simulink model "control_motor"  (R2024a)
settings: Solver=VariableStepAuto  StartTime=0.0  StopTime=1  FixedStep=0.0001  RelTol=1e-3
libraries: spsMosfetLib x8, spsGroundLib x2, eeTransforms x2, slpidlib x2, spsDCVoltageSourceLib x1, spsStepperMotorLib x1, spsVoltageMeasurementLib x1, spsTriangleGeneratorLib x1, sps_lib x1
settings Model: Creator=Damian  LastModifiedBy=PC
settings SolverCC: MaxConsecutiveZCs=100  MaxConsecutiveMinStep=10000  AllowMultiTaskInputOutput=on  ZeroCrossControl=EnableAll
settings ModelReferenceCC: ModelReferenceMinAlgLoopOccurrences=on

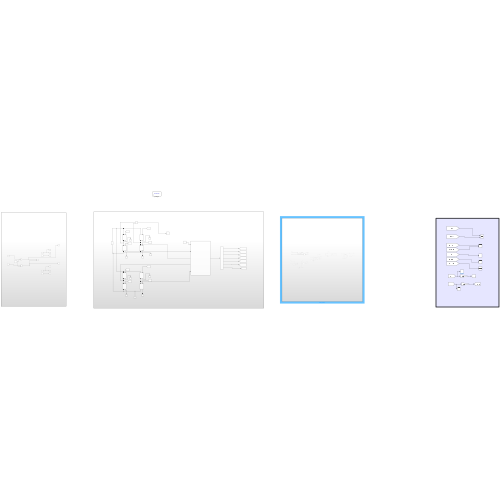
[thumbnail: Simulink's stored preview of the top-level diagram]
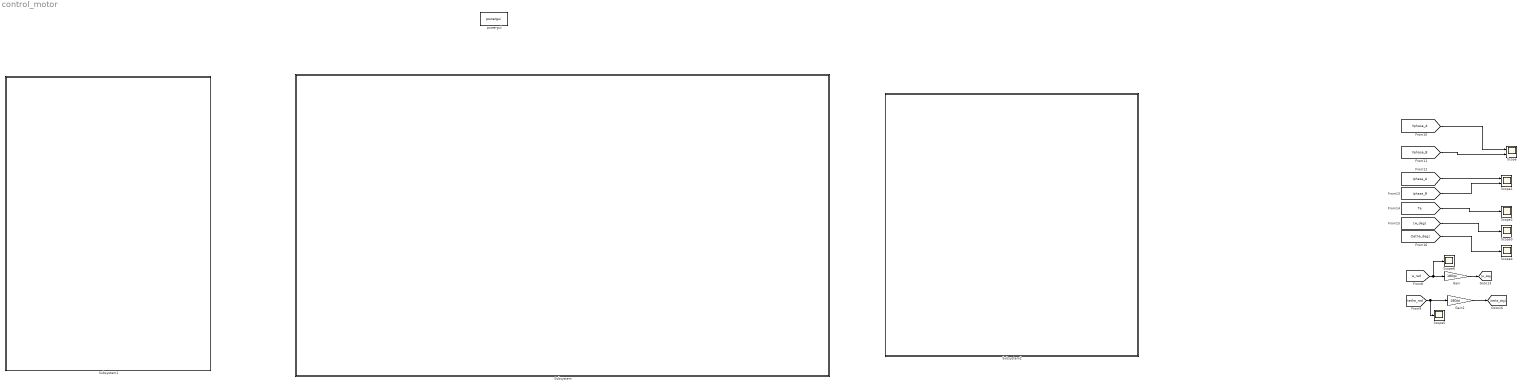
== system control_motor ==
  Gain : Gain  Gain=180/pi
  Gain1 : Gain  Gain=180/pi
  Scope : Scope  NumInputPorts=2
  Scope1 : Scope  NumInputPorts=2
  Scope{2..6} (5 alike) : Scope
  Subsystem : Subsystem
  Subsystem1 : Subsystem
  Subsystem2 : Subsystem
  powergui : sps_lib/powergui  Priority=1  SimulationMode=Continuous  SampleTime=1e-1  frequency=60  Iterations=50  frequencyindice=0  Pbase=100e6  ErrMax=1e-4  UnitsV=kV  UnitsW=MW  buscounter=0  FunctionMessages=off  echomessages=off  EnableUseOfTLC=off  CurrentSourceSwitches=off  DisableSnubberDevices=off  DisableRonSwitches=off  DisableVfSwitches=off  DisplayEquations=off  AutomaticDiscreteSolvers=off  SolverType=Tustin/Backward Euler (TBE)  Interpol=off  ExternalGateDelay=off  methode=off  Ts=100  x0status=blocks  SPID=on  SwTol=0  HookPort=off  NonlinearTolerance=1e-4  nMaxIteration=100  ContinueOnMaxIteration=off  RestoreLinks=warning  ResistiveCurrentMeasurement=off  Frange=[0:2:500]  Ylog=off  Xlog=on  ShowGrid=off  save=off  variable=ZData  structure=0  ZoomFFT=off  StartTime=0.0  cycles=1  DisplayStyle=1  fundamental=60  FreqAxis=off  MaxFrequency=1000  frequencyindicesteady=1  RmsSteady=1  display=off
  wires:
  [w_rad] -> Scope6/1, Gain/1
  Gain/1 -> [w_deg]
  [tetha_rad] -> Scope5/1, Gain1/1
  Gain1/1 -> [tetha_deg]
  [Vphase_A] -> Scope/1
  [Vphase_B] -> Scope/2
  [Iphase_A] -> Scope1/1
  [Iphase_B] -> Scope1/2
  [Te] -> Scope2/1
  [w_deg] -> Scope3/1
  [tetha_deg] -> Scope4/1

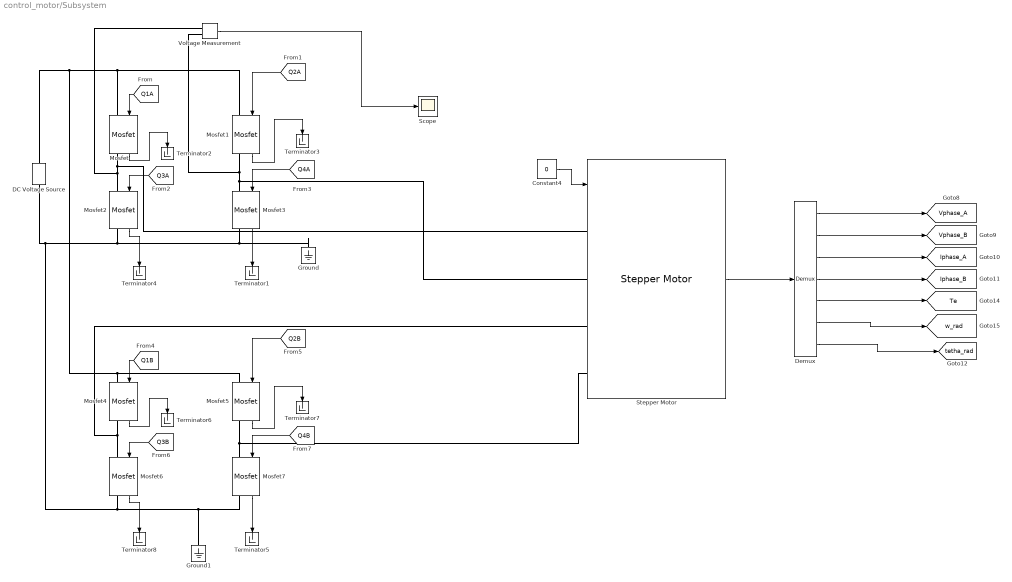
== system control_motor/Subsystem ==
  Constant4 : Constant  Value=0
  DC Voltage Source : spsDCVoltageSourceLib/DC Voltage Source  Amplitude=12  Measurements=None
  Demux : Demux  Outputs=7
  Ground : spsGroundLib/Ground  LConnTagsString=a
  Ground1 : spsGroundLib/Ground  LConnTagsString=a
  Mosfet{,1..7} (8 alike) : spsMosfetLib/Mosfet  Ron=0.1  Lon=0  Rd=0.01  Vfd=0  IC=0  Rs=1e5  Cs=inf  Measurements=on
  Scope : Scope
  Stepper Motor : spsStepperMotorLib/Stepper Motor  MotorType=Permanent-magnet / Hybrid  NumberOfPhases_1=2  NumberOfPhases_2=3  PresetModel_1=<empty>  PresetModel_2=<empty>  L=6e-3  Lmax=10e-3  Lmin=2e-3  R=3.4  Step_angle=1.8  Psim=0.04  Tdm=0.018  J=0.0000047  B=0  w0=0  pos0=0  TsPowergui=0  TsBlock=-1
      settings: LibrarySourceBlock=sps_lib/Electrical Machines/Stepper Motor
  Terminator{1..8} (8 alike) : Terminator
  Voltage Measurement : spsVoltageMeasurementLib/Voltage Measurement  PhasorSimulation=off  OutputType=Complex  PSBequivalent=0
  tag scope: Iphase_A=global, Iphase_B=global, Te=global, Vphase_A=global, Vphase_B=global, tetha_rad=global, w_rad=global
  wires:
  Demux/7 -> [tetha_rad]
  [Q3A] -> Mosfet2/1
  Mosfet7/1 -> Terminator5/1
  Demux/5 -> [Te]
  [Q2A] -> Mosfet1/1
  [Q4B] -> Mosfet7/1
  Mosfet1/1 -> Terminator3/1
  Demux/1 -> [Vphase_A]
  [Q4A] -> Mosfet3/1
  Demux/6 -> [w_rad]
  Mosfet4/1 -> Terminator6/1
  [Q1A] -> Mosfet/1
  Constant4/1 -> Stepper Motor/1
  [Q3B] -> Mosfet6/1
  [Q1B] -> Mosfet4/1
  Demux/4 -> [Iphase_B]
  Stepper Motor/1 -> Demux/1
  Mosfet2/1 -> Terminator4/1
  Mosfet/1 -> Terminator2/1
  Mosfet3/1 -> Terminator1/1
  [Q2B] -> Mosfet5/1
  Mosfet5/1 -> Terminator7/1
  Mosfet6/1 -> Terminator8/1
  Demux/2 -> [Vphase_B]
  Demux/3 -> [Iphase_A]
  Voltage Measurement/1 -> Scope/1
  connections:
  Mosfet6/RConn1 -- DC Voltage Source/LConn1 -- Ground/LConn1 -- Mosfet3/RConn1 -- Mosfet2/RConn1 -- Ground1/LConn1 -- Mosfet7/RConn1
  DC Voltage Source/RConn1 -- Mosfet5/LConn1 -- Mosfet4/LConn1 -- Mosfet1/LConn1 -- Mosfet/LConn1
  Mosfet/RConn1 -- Stepper Motor/LConn1 -- Voltage Measurement/LConn1 -- Mosfet2/LConn1
  Mosfet3/LConn1 -- Voltage Measurement/LConn2 -- Mosfet1/RConn1 -- Stepper Motor/LConn2
  Mosfet4/RConn1 -- Mosfet6/LConn1 -- Stepper Motor/LConn3
  Mosfet7/LConn1 -- Stepper Motor/LConn4 -- Mosfet5/RConn1

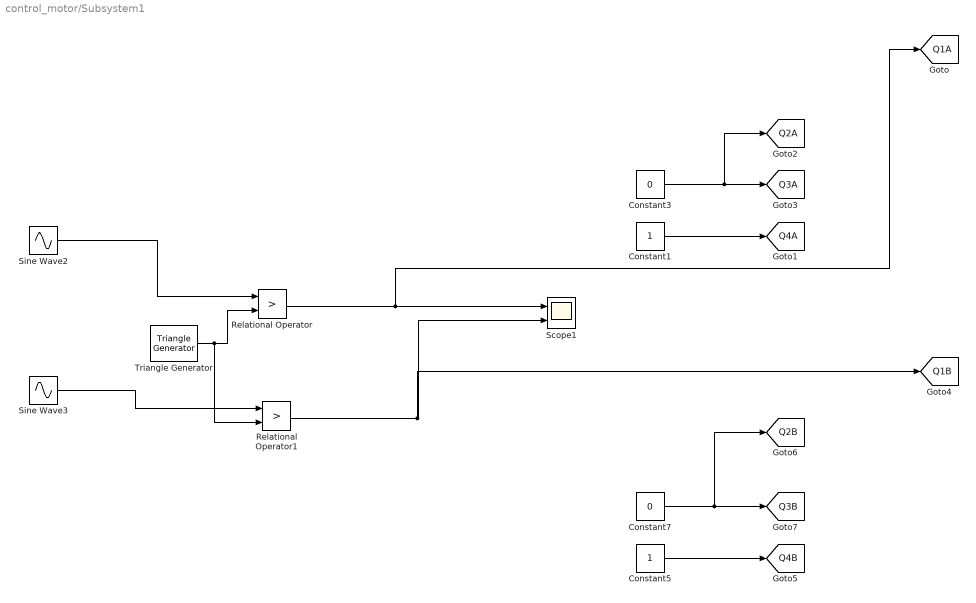
== system control_motor/Subsystem1 ==
  Constant1 : Constant
  Constant3 : Constant  Value=0
  Constant5 : Constant
  Constant7 : Constant  Value=0
  Relational Operator : RelationalOperator  Operator=>  RndMeth=Simplest  InputSameDT=off
  Relational Operator1 : RelationalOperator  Operator=>  RndMeth=Simplest  InputSameDT=off
  Scope1 : Scope  NumInputPorts=2
  Sine Wave2 : Sin  Frequency=2*pi*50  SampleTime=0
  Sine Wave3 : Sin  Amplitude=1.5  Frequency=2*pi*50  Phase=pi/2  SampleTime=0
  Triangle Generator : spsTriangleGeneratorLib/Triangle Generator  Freq=1e4  Phase=0  Ts=0
  tag scope: Q1A=global, Q1B=global, Q2A=global, Q2B=global, Q3A=global, Q3B=global, Q4A=global, Q4B=global
  wires:
  Constant3/1 -> [Q2A], [Q3A]
  Constant7/1 -> [Q2B], [Q3B]
  Constant5/1 -> [Q4B]
  Constant1/1 -> [Q4A]
  Relational Operator/1 -> [Q1A], Scope1/1
  Triangle Generator/1 -> Relational Operator1/2, Relational Operator/2
  Relational Operator1/1 -> [Q1B], Scope1/2
  Sine Wave2/1 -> Relational Operator/1
  Sine Wave3/1 -> Relational Operator1/1

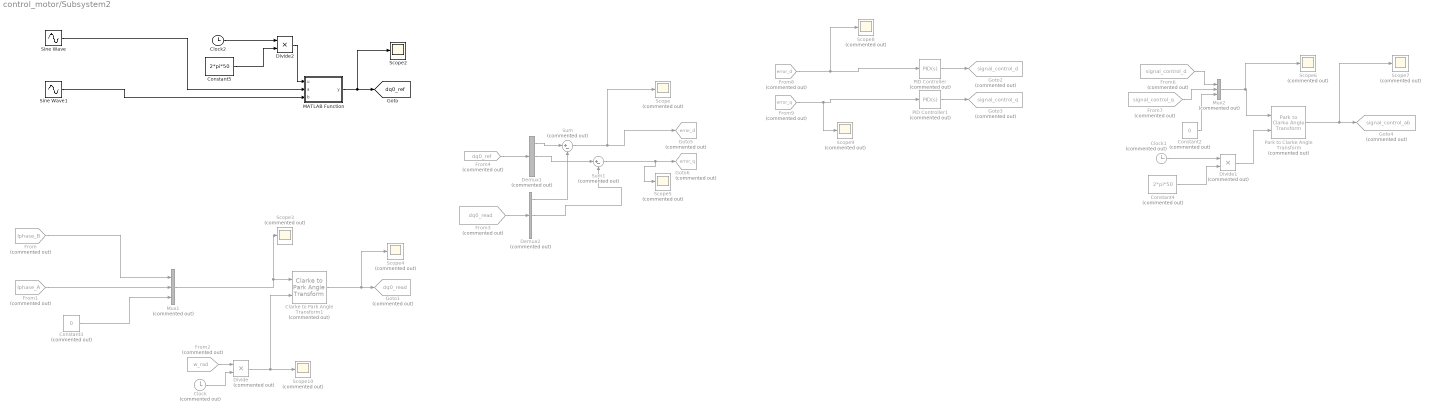
== system control_motor/Subsystem2 ==
  Clarke to Park Angle Transform1 : eeTransforms/Clarke to Park Angle Transform  Commented=on  AxisAlignment=D-axis
      settings: LibrarySourceBlock=|
      | ee_sl_lib/Mathematical
      | Transforms/Clarke to Park
      | Angle Transform
  Clock : Clock  Commented=on
  Clock1 : Clock  Commented=on
  Clock2 : Clock
  Constant2 : Constant  Commented=on  Value=0
  Constant3 : Constant  Commented=on  Value=0
  Constant4 : Constant  Commented=on  Value=2*pi*50
  Constant5 : Constant  Value=2*pi*50
  Demux1 : Demux  Commented=on  Outputs=3
  Demux2 : Demux  Commented=on  Outputs=3
  Divide : Product  Commented=on  Inputs=**
  Divide1 : Product  Commented=on  Inputs=**
  Divide2 : Product  Inputs=**
  From : From  Commented=on  GotoTag=Iphase_B  TagVisibility=global
  From1 : From  Commented=on  GotoTag=Iphase_A  TagVisibility=global
  From2 : From  Commented=on  GotoTag=w_rad  TagVisibility=global
  From3 : From  Commented=on  GotoTag=dq0_read  TagVisibility=global
  From4 : From  Commented=on  GotoTag=dq0_ref  TagVisibility=global
  From6 : From  Commented=on  GotoTag=signal_control_d  TagVisibility=global
  From7 : From  Commented=on  GotoTag=signal_control_q  TagVisibility=global
  From8 : From  Commented=on  GotoTag=error_d  TagVisibility=global
  From9 : From  Commented=on  GotoTag=error_q  TagVisibility=global
  Goto1 : Goto  Commented=on  GotoTag=dq0_read  TagVisibility=global
  Goto2 : Goto  Commented=on  GotoTag=signal_control_d  TagVisibility=global
  Goto3 : Goto  Commented=on  GotoTag=signal_control_q  TagVisibility=global
  Goto4 : Goto  Commented=on  GotoTag=signal_control_ab  TagVisibility=global
  Goto5 : Goto  Commented=on  GotoTag=error_d  TagVisibility=global
  Goto6 : Goto  Commented=on  GotoTag=error_q  TagVisibility=global
  MATLAB Function : MATLAB Function  TreatAsAtomicUnit=on
  Mux1 : Mux  Commented=on  Inputs=3
  Mux2 : Mux  Commented=on  Inputs=3
  PID Controller : slpidlib/PID Controller  Commented=on  Controller=PID  Form=Parallel  TimeDomain=Continuous-time  UseExternalTs=off  SampleTime=-1  IntegratorMethod=Forward Euler  FilterMethod=Forward Euler  ControllerParametersSource=internal  P=1  I=1  UseKiTs=off  D=0  UseExternalDerivativeSource=off  N=100  UseFilter=on  TunerSelectOption=Transfer Function Based (PID Tuner App)  InitialConditionSource=internal  InitialConditionForIntegrator=0  InitialConditionForFilter=0  DifferentiatorICPrevScaledInput=0  ExternalReset=none  TrackingMode=off  Kt=1  LimitOutput=on  SatLimitsSource=internal  UpperSaturationLimit=1  LowerSaturationLimit=0  LinearizeAsGain=on  AntiWindupMode=none  Kb=1  LimitIntegrator=on  UpperIntegratorSaturationLimit=1  LowerIntegratorSaturationLimit=0  POutMin=[]  POutMax=[]  IOutMin=[]  IOutMax=[]  DOutMin=[]  DOutMax=[]  NOutMin=[]  NOutMax=[]  SumOutMin=[]  SumOutMax=[]  SaturationOutMin=[]  SaturationOutMax=[]  PParamMin=[]  PParamMax=[]  IParamMin=[]  IParamMax=[]  DParamMin=[]  DParamMax=[]  NParamMin=[]  NParamMax=[]  KbParamMin=[]  KbParamMax=[]  KtParamMin=[]  KtParamMax=[]  KbOutMin=[]  KbOutMax=[]  KtOutMin=[]  KtOutMax=[]  IntegratorOutMin=[]  IntegratorOutMax=[]  FilterOutMin=[]  FilterOutMax=[]  SumI1OutMin=[]  SumI1OutMax=[]  SumI2OutMin=[]  SumI2OutMax=[]  SumI3OutMin=[]  SumI3OutMax=[]  SumI4OutMin=[]  SumI4OutMax=[]  SumDOutMin=[]  SumDOutMax=[]  DifferentiatorOutMin=[]  DifferentiatorOutMax=[]  FilterDiffOutCoefMin=[]  FilterDiffOutCoefMax=[]  ReciprocalOutMin=[]  ReciprocalOutMax=[]  SumDenOutMin=[]  SumDenOutMax=[]  SumNumOutMin=[]  SumNumOutMax=[]  DivideOutMin=[]  DivideOutMax=[]  UdiffTsProdOutMin=[]  UdiffTsProdOutMax=[]  NTsProdOutMin=[]  NTsProdOutMax=[]  UintegralTsProdOutMin=[]  UintegralTsProdOutMax=[]  UngainTsProdOutMin=[]  UngainTsProdOutMax=[]  ClampingZeroOutDataTypeStr=Inherit: Inherit via back propagation  ClampingZeroOutMin=[]  ClampingZeroOutMax=[]  FilterDenConstantOutDataTypeStr=Inherit: Inherit via back propagation  FilterDenConstantOutMin=[]  FilterDenConstantOutMax=[]  PCopyOutDataTypeStr=Inherit: Inherit via back propagation  PCopyOutMin=[]  PCopyOutMax=[]  NCopyOutDataTypeStr=Inherit: Inherit via back propagation  NCopyOutMin=[]  NCopyOutMax=[]  IntegratorContinuousStateAttributes=''  IntegratorStateMustResolveToSignalObject=off  IntegratorRTWStateStorageClass=Auto  FilterContinuousStateAttributes=''  FilterStateMustResolveToSignalObject=off  FilterRTWStateStorageClass=Auto  ParallelPVariant=InternalParameters  IdealPVariant=Disabled  IVariant=InternalParameters  DVariant=InternalParameters  IntegratorVariant=Continuous  SatVariant=Enabled  AWVariant=Passthrough  PCopyVariant=Disabled  TRVariant=Disabled  FdbkBlocksVariant=Forward  IdealPFdbkVariant=Disabled  SatFdbkVariant=Disabled  DerivativeFilterVariant=ContFilter  NVariant=InternalParameters  NCopyVariant=Disabled  FilterICVariant=InternalICsFilter  IntegratorICVariant=InternalICs  ExternalResetVariant=Disabled  TRSumVariant=Passthrough  SumFdbkVariant=Disabled  SumVariant=Sum_PID  TsampFilterVariant=InternalTs  TsampNgainVariant=Passthrough  TsampIntegralVariant=Disabled_SignalSpec  ExternalSaturationOutDataTypeStr=Inherit: Same as second input  DerivativeSourceVariant=ErrorSignal
  PID Controller1 : slpidlib/PID Controller  Commented=on  Controller=PID  Form=Parallel  TimeDomain=Continuous-time  UseExternalTs=off  SampleTime=-1  IntegratorMethod=Forward Euler  FilterMethod=Forward Euler  ControllerParametersSource=internal  P=1  I=1  UseKiTs=off  D=0  UseExternalDerivativeSource=off  N=100  UseFilter=on  TunerSelectOption=Transfer Function Based (PID Tuner App)  InitialConditionSource=internal  InitialConditionForIntegrator=0  InitialConditionForFilter=0  DifferentiatorICPrevScaledInput=0  ExternalReset=none  TrackingMode=off  Kt=1  LimitOutput=on  SatLimitsSource=internal  UpperSaturationLimit=1  LowerSaturationLimit=0  LinearizeAsGain=on  AntiWindupMode=none  Kb=1  LimitIntegrator=on  UpperIntegratorSaturationLimit=1  LowerIntegratorSaturationLimit=0  POutMin=[]  POutMax=[]  IOutMin=[]  IOutMax=[]  DOutMin=[]  DOutMax=[]  NOutMin=[]  NOutMax=[]  SumOutMin=[]  SumOutMax=[]  SaturationOutMin=[]  SaturationOutMax=[]  PParamMin=[]  PParamMax=[]  IParamMin=[]  IParamMax=[]  DParamMin=[]  DParamMax=[]  NParamMin=[]  NParamMax=[]  KbParamMin=[]  KbParamMax=[]  KtParamMin=[]  KtParamMax=[]  KbOutMin=[]  KbOutMax=[]  KtOutMin=[]  KtOutMax=[]  IntegratorOutMin=[]  IntegratorOutMax=[]  FilterOutMin=[]  FilterOutMax=[]  SumI1OutMin=[]  SumI1OutMax=[]  SumI2OutMin=[]  SumI2OutMax=[]  SumI3OutMin=[]  SumI3OutMax=[]  SumI4OutMin=[]  SumI4OutMax=[]  SumDOutMin=[]  SumDOutMax=[]  DifferentiatorOutMin=[]  DifferentiatorOutMax=[]  FilterDiffOutCoefMin=[]  FilterDiffOutCoefMax=[]  ReciprocalOutMin=[]  ReciprocalOutMax=[]  SumDenOutMin=[]  SumDenOutMax=[]  SumNumOutMin=[]  SumNumOutMax=[]  DivideOutMin=[]  DivideOutMax=[]  UdiffTsProdOutMin=[]  UdiffTsProdOutMax=[]  NTsProdOutMin=[]  NTsProdOutMax=[]  UintegralTsProdOutMin=[]  UintegralTsProdOutMax=[]  UngainTsProdOutMin=[]  UngainTsProdOutMax=[]  ClampingZeroOutDataTypeStr=Inherit: Inherit via back propagation  ClampingZeroOutMin=[]  ClampingZeroOutMax=[]  FilterDenConstantOutDataTypeStr=Inherit: Inherit via back propagation  FilterDenConstantOutMin=[]  FilterDenConstantOutMax=[]  PCopyOutDataTypeStr=Inherit: Inherit via back propagation  PCopyOutMin=[]  PCopyOutMax=[]  NCopyOutDataTypeStr=Inherit: Inherit via back propagation  NCopyOutMin=[]  NCopyOutMax=[]  IntegratorContinuousStateAttributes=''  IntegratorStateMustResolveToSignalObject=off  IntegratorRTWStateStorageClass=Auto  FilterContinuousStateAttributes=''  FilterStateMustResolveToSignalObject=off  FilterRTWStateStorageClass=Auto  ParallelPVariant=InternalParameters  IdealPVariant=Disabled  IVariant=InternalParameters  DVariant=InternalParameters  IntegratorVariant=Continuous  SatVariant=Enabled  AWVariant=Passthrough  PCopyVariant=Disabled  TRVariant=Disabled  FdbkBlocksVariant=Forward  IdealPFdbkVariant=Disabled  SatFdbkVariant=Disabled  DerivativeFilterVariant=ContFilter  NVariant=InternalParameters  NCopyVariant=Disabled  FilterICVariant=InternalICsFilter  IntegratorICVariant=InternalICs  ExternalResetVariant=Disabled  TRSumVariant=Passthrough  SumFdbkVariant=Disabled  SumVariant=Sum_PID  TsampFilterVariant=InternalTs  TsampNgainVariant=Passthrough  TsampIntegralVariant=Disabled_SignalSpec  ExternalSaturationOutDataTypeStr=Inherit: Same as second input  DerivativeSourceVariant=ErrorSignal
  Park to Clarke Angle Transform : eeTransforms/Park to Clarke Angle Transform  Commented=on  AxisAlignment=Q-axis
      settings: LibrarySourceBlock=|
      | ee_sl_lib/Mathematical
      | Transforms/Park to Clarke
      | Angle Transform
  Scope{,3..10} (9 alike) : Scope  Commented=on
  Scope2 : Scope
  Sine Wave : Sin  Amplitude=1.5  Frequency=2*pi*50  Phase=pi/2  SampleTime=0
  Sine Wave1 : Sin  Amplitude=1.5  Frequency=2*pi*50  SampleTime=0
  Sum : Sum  Commented=on  Inputs=|+-
  Sum1 : Sum  Commented=on  Inputs=|+-
  tag scope: dq0_ref=global
  wires:
  Sine Wave1/1 -> MATLAB Function/3(b)
  Sine Wave/1 -> MATLAB Function/2(a)
  From/1 -> Mux1/1
  From1/1 -> Mux1/2
  Mux1/1 -> Scope3/1, Clarke to Park Angle Transform1/1
  Constant3/1 -> Mux1/3
  Clarke to Park Angle Transform1/1 -> Goto1/1, Scope4/1
  From4/1 -> Demux1/1
  PID Controller1/1 -> Goto3/1
  PID Controller/1 -> Goto2/1
  From6/1 -> Mux2/1
  From7/1 -> Mux2/2
  Mux2/1 -> Scope6/1, Park to Clarke Angle Transform/1
  Park to Clarke Angle Transform/1 -> Scope7/1, Goto4/1
  Constant2/1 -> Mux2/3
  Sum/1 -> Scope/1, Goto5/1
  From8/1 -> Scope8/1, PID Controller/1
  From9/1 -> Scope9/1, PID Controller1/1
  From3/1 -> Demux2/1
  Demux1/1 -> Sum/1
  Demux2/1 -> Sum/2
  Demux1/2 -> Sum1/1
  Sum1/1 -> Scope5/1, Goto6/1
  Demux2/2 -> Sum1/2
  Divide1/1 -> Park to Clarke Angle Transform/2
  Constant4/1 -> Divide1/2
  Clock1/1 -> Divide1/1
  Clock2/1 -> Divide2/1
  Constant5/1 -> Divide2/2
  From2/1 -> Divide/1
  Clock/1 -> Divide/2
  Divide/1 -> Scope10/1, Clarke to Park Angle Transform1/2
  MATLAB Function/1(y) -> Scope2/1, [dq0_ref]
  Divide2/1 -> MATLAB Function/1(u)

== matlab function control_motor/Subsystem2/MATLAB Function ==
  data: u input; y output; a input; b input
function y = fcn(u,a,b)
    M = [cos(2*u) sin(2*u); -sin(2*u) cos(2*u)];
    y = M * [a; b];
end
